simulink model "EnvelopeDetector"  (Simulink 7.1)
settings: Solver=ode23t  StartTime=0.0  StopTime=0.1  FixedStep=1e-6  RelTol=1e-3
undefined symbols (not defined in the file): C, fs, R
libraries: powerlib x11, powerlib_extras x3, simulink x1, simulink_extras x1
settings Model: Creator=Ugo.Pattacini  LastModifiedBy=Carchesion
settings DataIOCC: LimitDataPoints=off  SaveOutput=off  SignalLogging=off  SaveTime=off
settings DebuggingCC: SaveWithParameterizedLinksMsg=none  SignalResolutionControl=TryResolveAllWithWarning  MultiTaskDSMMsg=warning  MultiTaskCondExecSysMsg=none
settings RTWCC: IncludeERTFirstTime=on
settings GRTTargetCC: TargetFcnLib=ansi_tfl_tmw.mat

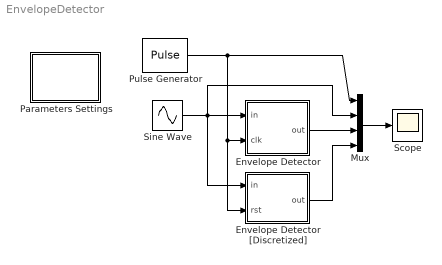
== system EnvelopeDetector ==
  Envelope Detector : Subsystem  mask{R=R, C=C}
      mask prompts: R "Resistance (Ohm):"; C "Capacitance (F):"
  Envelope Detector [Discretized] : Subsystem  mask(Envelope Detector){tau=R*C, Ts=1e-6}
      mask prompts: tau "tau (s):"; Ts "Sample time (s):"
      mask help: Implement an Envelope Detection
  Mux : Mux
  Parameters Settings : Subsystem  mask(Parametes Settings.){R=1e3, C=1e-6}
      mask prompts: R "Resistance (Ohm):"; C "Capacitance (F):"
      mask help: Parametes Settings.
      mask init:
      | str=sprintf('R=%g\nC=%g',R,C);
      | 
      | assignin('base','R',R);
      | assignin('base','C',C);
      mask Display: disp(str);
  Pulse Generator : DiscretePulseGenerator  PulseType=Time based  Period=0.01  PulseWidth=50  SampleTime=(1/fs)/10
  Scope : Scope
      settings: TimeRange=0.25  YMin=-1.1  YMax=1.1
  Sine Wave : Sin  Frequency=2*pi*500  SampleTime=0
  wires:
  Pulse Generator/1 -> Envelope Detector/2(clk), Envelope Detector [Discretized]/2(rst), Mux/1
  Sine Wave/1 -> Envelope Detector/1(in), Envelope Detector [Discretized]/1(in), Mux/2
  Envelope Detector/1(out) -> Mux/3
  Envelope Detector [Discretized]/1(out) -> Mux/4
  Mux/1 -> Scope/1

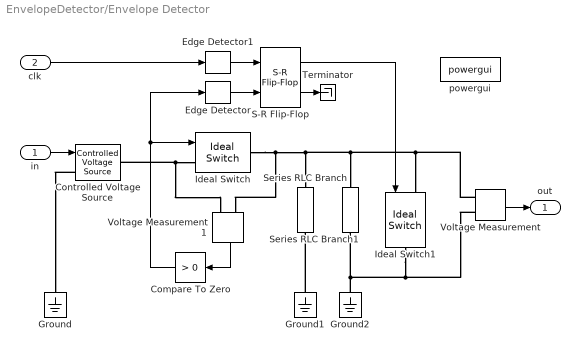
== system EnvelopeDetector/Envelope Detector ==
  in : Inport  OutDataType=sfix(16)  OutScaling=2^0
  clk : Inport  Port=2  OutDataType=sfix(16)  OutScaling=2^0
  Compare To Zero : simulink/Logic and Bit Operations/Compare To Zero  Orientation=left  SystemSampleTime=-1  relop=>  LogicOutDataTypeMode=boolean  ZeroCross=off
  Controlled Voltage Source : powerlib/Electrical Sources/Controlled Voltage Source  DialogController=POWERSYS.PowerSysDialog  SystemSampleTime=-1  Initialize=off  Source_Type=AC  Amplitude=0  Phase=0  Frequency=0  Measurements=None
  Edge Detector : powerlib_extras/Control  Blocks/Edge Detector  DialogController=POWERSYS.PowerSysDialog  SystemSampleTime=-1  model=Rising  ic=0
  Edge Detector1 : powerlib_extras/Control  Blocks/Edge Detector  DialogController=POWERSYS.PowerSysDialog  SystemSampleTime=-1  model=Either  ic=0
  Ground : powerlib/Elements/Ground  Orientation=down  DialogController=POWERSYS.PowerSysDialog  PhysicalDomain=powersysdomain  SubClassName=unknown  LeftPortType=p1  RightPortType=p1  LConnTagsString=a
  Ground1 : powerlib/Elements/Ground  Orientation=down  DialogController=POWERSYS.PowerSysDialog  PhysicalDomain=powersysdomain  SubClassName=unknown  LeftPortType=p1  RightPortType=p1  LConnTagsString=a
  Ground2 : powerlib/Elements/Ground  Orientation=down  DialogController=POWERSYS.PowerSysDialog  PhysicalDomain=powersysdomain  SubClassName=unknown  LeftPortType=p1  RightPortType=p1  LConnTagsString=a
  Ideal Switch : powerlib/Power Electronics/Ideal Switch  DialogController=POWERSYS.PowerSysDialog  SystemSampleTime=-1  Ron=0.001  Lon=0  IC=1  Rs=inf  Cs=inf  Measurements=off
  Ideal Switch1 : powerlib/Power Electronics/Ideal Switch  Orientation=down  DialogController=POWERSYS.PowerSysDialog  SystemSampleTime=-1  Ron=1  Lon=0  IC=0  Rs=inf  Cs=inf  Measurements=off
  S-R Flip-Flop : simulink_extras/Flip Flops/S-R Flip-Flop  SystemSampleTime=-1  initial_condition=0
  Series RLC Branch : powerlib/Elements/Series RLC Branch  Orientation=down  DialogController=POWERSYS.PowerSysDialog  PhysicalDomain=powersysdomain  SubClassName=unknown  LeftPortType=p1  RightPortType=p1  LConnTagsString=__new0  RConnTagsString=__new0  BranchType=R  Resistance=R  Inductance=1e-3  SetiL0=off  InitialCurrent=0  Capacitance=1e-6  Setx0=off  InitialVoltage=0  Measurements=None
  Series RLC Branch1 : powerlib/Elements/Series RLC Branch  Orientation=down  DialogController=POWERSYS.PowerSysDialog  PhysicalDomain=powersysdomain  SubClassName=unknown  LeftPortType=p1  RightPortType=p1  LConnTagsString=__new0  RConnTagsString=__new0  BranchType=C  Resistance=1  Inductance=1e-3  SetiL0=off  InitialCurrent=0  Capacitance=C  Setx0=off  InitialVoltage=0  Measurements=None
  Terminator : Terminator
  Voltage Measurement : powerlib/Measurements/Voltage Measurement  DialogController=POWERSYS.PowerSysDialog  SystemSampleTime=-1  PhasorSimulation=off  OutputType=Complex  PSBequivalent=0
  Voltage Measurement1 : powerlib/Measurements/Voltage Measurement  Orientation=down  DialogController=POWERSYS.PowerSysDialog  SystemSampleTime=-1  PhasorSimulation=off  OutputType=Complex  PSBequivalent=0
  powergui : powerlib/powergui  SystemSampleTime=-1  SimulationMode=Continuous  SampleTime=1e-6  frequency=60  SPID=off  SwTol=0  Interpol=off  x0status=blocks  echomessages=off  HookPort=off  FunctionMessages=off  EnableUseOfTLC=off  RestoreLinks=warning  frequencyindice=0  Frange=[0:2:500]  Ylog=off  Xlog=on  ShowGrid=off  save=off  variable=ZData  ZoomFFT=on  StartTime=0.0  cycles=1  DisplayStyle=1  fundamental=60  FreqAxis=off  MaxFrequency=1000  frequencyindicesteady=1  RmsSteady=1  display=off  Ts=0  methode=off
  out : Outport  OutDataType=sfix(16)  OutScaling=2^0
  wires:
  Voltage Measurement1/1 -> Compare To Zero/1
  Compare To Zero/1 -> Edge Detector/1, Ideal Switch/1
  in/1 -> Controlled Voltage Source/1
  Voltage Measurement/1 -> out/1
  clk/1 -> Edge Detector1/1
  Edge Detector/1 -> S-R Flip-Flop/2
  Edge Detector1/1 -> S-R Flip-Flop/1
  S-R Flip-Flop/2 -> Terminator/1
  S-R Flip-Flop/1 -> Ideal Switch1/1
  connections:
  Controlled Voltage Source/LConn1 -- Ground/LConn1
  Controlled Voltage Source/RConn1 -- Voltage Measurement1/LConn1 -- Ideal Switch/LConn1
  Ground1/LConn1 -- Series RLC Branch/RConn1
  Ground2/LConn1 -- Ideal Switch1/RConn1 -- Voltage Measurement/LConn2 -- Series RLC Branch1/RConn1
  Voltage Measurement/LConn1 -- Series RLC Branch1/LConn1 -- Ideal Switch/RConn1 -- Voltage Measurement1/LConn2 -- Series RLC Branch/LConn1 -- Ideal Switch1/LConn1

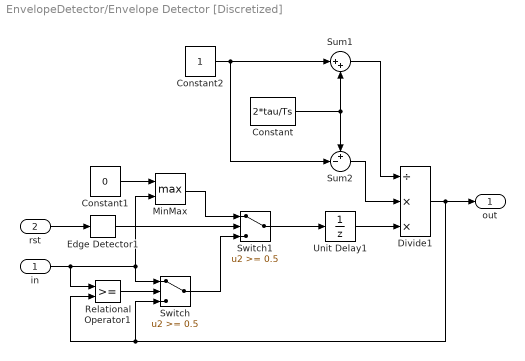
== system EnvelopeDetector/Envelope Detector [Discretized] ==
  in : Inport  OutDataType=sfix(16)  OutScaling=2^0
  rst : Inport  Port=2  OutDataType=sfix(16)  OutScaling=2^0
  Constant : Constant  Value=2*tau/Ts  OutDataType=sfix(16)  OutScaling=2^0
  Constant1 : Constant  Value=0  OutDataType=sfix(16)  OutScaling=2^0
  Constant2 : Constant  OutDataType=sfix(16)  OutScaling=2^0
  Divide1 : Product  Inputs=/**  OutDataType=sfix(16)  OutScaling=2^-10
  Edge Detector1 : powerlib_extras/Control  Blocks/Edge Detector  DialogController=POWERSYS.PowerSysDialog  SystemSampleTime=-1  model=Either  ic=0
  MinMax : MinMax  Function=max  Inputs=2  OutDataType=sfix(16)  OutScaling=2^0
  Relational Operator1 : RelationalOperator  LogicOutDataTypeMode=boolean  OutDataTypeStr=boolean
  Sum1 : Sum  Inputs=|++  OutDataType=sfix(16)  OutScaling=2^0
  Sum2 : Sum  Inputs=+-|  OutDataType=sfix(16)  OutScaling=2^0
  Switch : Switch  Threshold=0.5
  Switch1 : Switch  Threshold=0.5
  Unit Delay1 : UnitDelay  SampleTime=Ts
  out : Outport  OutDataType=sfix(16)  OutScaling=2^0
  wires:
  Constant/1 -> Sum1/2, Sum2/1
  Divide1/1 -> Relational Operator1/2, Switch/3, out/1
  in/1 -> Relational Operator1/1, Switch/1, MinMax/2
  Relational Operator1/1 -> Switch/2
  Unit Delay1/1 -> Divide1/3
  Sum2/1 -> Divide1/2
  Constant2/1 -> Sum1/1, Sum2/2
  Sum1/1 -> Divide1/1
  Switch/1 -> Switch1/3
  Switch1/1 -> Unit Delay1/1
  rst/1 -> Edge Detector1/1
  Edge Detector1/1 -> Switch1/2
  MinMax/1 -> Switch1/1
  Constant1/1 -> MinMax/1

== system EnvelopeDetector/Parameters Settings ==
